simulink model "AEL_simple_model_v02"  (R2022b)
settings: Solver=FixedStepAuto  StartTime=0.0  StopTime=1  FixedStep=0.001  RelTol=1e-3  EnableMultiTasking=on
settings Model: Creator=Kumar  LastModifiedBy=Kumar
settings SolverCC: AllowMultiTaskInputOutput=on
settings DebuggingCC: MaxConsecutiveZCsMsg=none  ModelReferenceExtraNoncontSigs=none

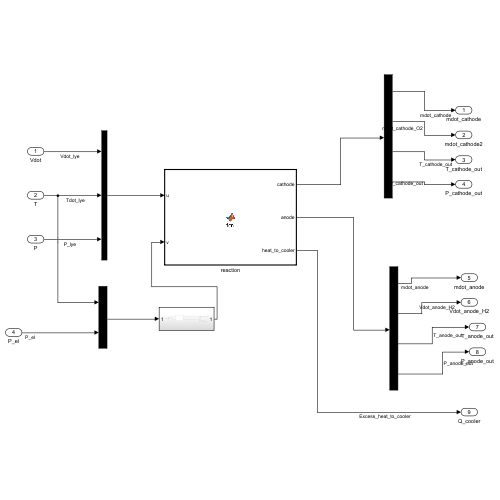
[thumbnail: Simulink's stored preview of the top-level diagram]
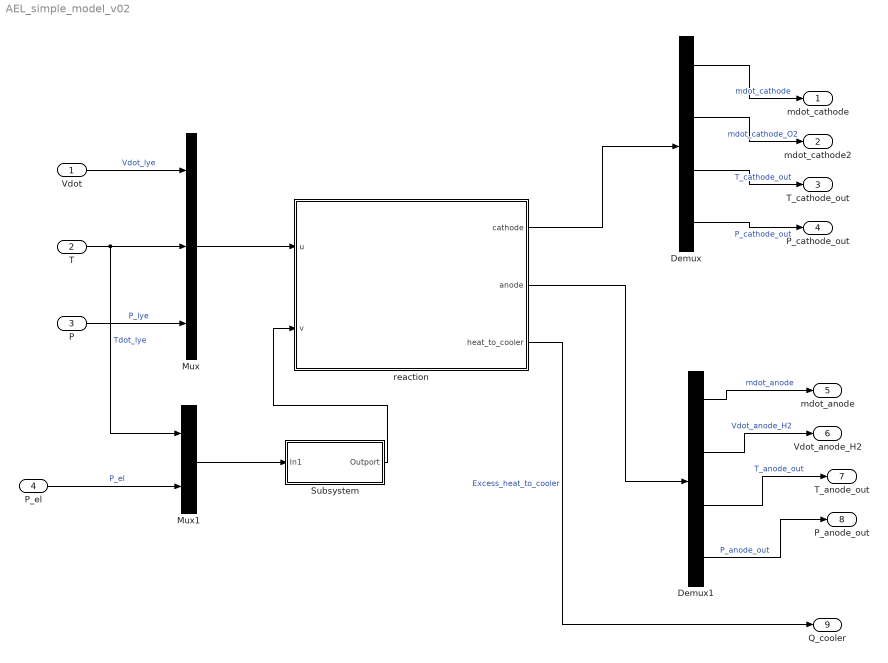
== system AEL_simple_model_v02 ==
  Vdot : Inport
  T : Inport  Port=2
  P : Inport  Port=3
  P_el : Inport  Port=4
  Demux : Demux
  Demux1 : Demux
  Mux : Mux  Inputs=3
  Mux1 : Mux  Inputs=2
  Subsystem : Subsystem
  reaction : MATLAB Function  TreatAsAtomicUnit=on
  mdot_cathode : Outport
  mdot_cathode2 : Outport  Port=2
  T_cathode_out : Outport  Port=3
  P_cathode_out : Outport  Port=4
  mdot_anode : Outport  Port=5
  Vdot_anode_H2 : Outport  Port=6
  T_anode_out : Outport  Port=7
  P_anode_out : Outport  Port=8
  Q_cooler : Outport  Port=9
  wires:
  Vdot/1 -> Mux/1  "Vdot_lye"
  Demux1/1 -> mdot_anode/1  "mdot_anode"
  T/1 -> Mux1/1, Mux/2  "Tdot_lye"
  Demux/1 -> mdot_cathode/1  "mdot_cathode"
  Mux/1 -> reaction/1(u)
  Demux1/2 -> Vdot_anode_H2/1  "Vdot_anode_H2"
  reaction/3(heat_to_cooler) -> Q_cooler/1  "Excess_heat_to_cooler"
  Mux1/1 -> Subsystem/1(In1)
  P/1 -> Mux/3  "P_lye"
  P_el/1 -> Mux1/2  "P_el"
  reaction/2(anode) -> Demux1/1
  Subsystem/1(Outport) -> reaction/2(v)
  reaction/1(cathode) -> Demux/1
  Demux/3 -> T_cathode_out/1  "T_cathode_out"
  Demux1/3 -> T_anode_out/1  "T_anode_out"
  Demux/4 -> P_cathode_out/1  "P_cathode_out"
  Demux/2 -> mdot_cathode2/1  "mdot_cathode_O2"
  Demux1/4 -> P_anode_out/1  "P_anode_out"

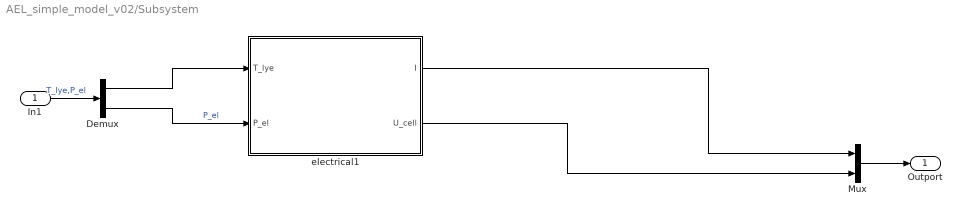
== system AEL_simple_model_v02/Subsystem ==
  In1 : Inport
  Demux : Demux  Outputs=2
  Mux : Mux  Inputs=2
  electrical1 : MATLAB Function  TreatAsAtomicUnit=on
  Outport : Outport
  wires:
  In1/1 -> Demux/1  "T_lye,P_el"
  Demux/1 -> electrical1/1(T_lye)
  Mux/1 -> Outport/1
  electrical1/1(I) -> Mux/1
  electrical1/2(U_cell) -> Mux/2
  Demux/2 -> electrical1/2(P_el)  "P_el"

== matlab function AEL_simple_model_v02/reaction ==
  data: u input; cathode output; anode output; heat_to_cooler output; v input
function [cathode, anode, heat_to_cooler] = fcn(u,v)

% Modelling assumptions: 
% 30% KOH solution
% Parameters

MwtH2 = 2.0; % Molecular weight of Hydrogen kg/kmol
MwtO2 = 32.0; % Molecular weight of Oxygen kg/kmol
MwtH2O = 18.0; % Molecular weight of water kg/kmol
z_value = 2; % Number of electrons transferred 
Farad = 96485000; % C/K mole Faraday's constant
param_d1 = -3.12996*10^-6; % Parameter from the polarization curve ohm m²
param_d2 = 4.47137 * 10^-7; % Parameter from the polarization curve ohm m² bar-1
A_electrode =  0.25; % Please note that the unit for current density is in m²
rho_lye = 1290; % Density of the KOH solution in kg/m³ --> Assumed constant 
n_c = 21; % No.of cells
R = 8.3144; % Gas constant KJ/KmolK
del_H0 = 286000; % standard enthalpy of reaction KJ/Kmol
T_amb = 298.15; % Ambient temperature - 25°C
Cp_lye = 4.2; % KJ/Kg K Specific heat capacity of lye --> assumed as that of water 

% Inputs

Vdot_lye = u(1) /(1000*3600); % volumetric flow of lye --> lph --> m³/s
T_lye = u(2); %353.75; % Temperature of lye K 
P_lye = u(3); %7.1  % Pressure of lye bar

I = v(1); % calculated current A/cm²
U_cell= v(2); % calculated voltage of cell V

% Equations

% Total electrode area
A = n_c * A_electrode; % m2 --> cm² needed

% Minimum reversible voltage
%U_rev = del_G/(z_value * Farad);

% Efficiency of the cell
yeta_f = 0.5; %(I/A)^2/(param_f1 + (I/A)^2) * param_f2; %0.86; %
% Mass balance
% Lye input at anode
mdot_anode_H2O = (Vdot_lye * rho_lye * 0.7) / 2; % kg/s
mdot_anode_KOH = (Vdot_lye * rho_lye * 0.3) / 2; % kg/s
ndot_anode_H2O = mdot_anode_H2O / MwtH2O; % kmol/s

% Lye input at cathode
mdot_cathode_H2O = (Vdot_lye * rho_lye* 0.7) / 2;  % kg/s
mdot_cathode_KOH = (Vdot_lye * rho_lye * 0.3) / 2;  % kg/s
ndot_cathode_H2O = mdot_cathode_H2O / MwtH2O;  % kmol/s

% Hydrogen produced at anode
ndot_anode_H2 = yeta_f * I /(z_value * Farad);% kmol/s
mdot_anode_H2 = ndot_anode_H2 * MwtH2; % kg/s
Vdot_anode_H2 = ndot_anode_H2 * 22.414; % Nm³/s

% Water going out of anode
ndot_anode_H2O_out = ndot_anode_H2O - ndot_anode_H2;% kmol/s
mdot_anode_H2O_out = ndot_anode_H2O_out * MwtH2O;% kg/s

% Oxygen produced at cathode
ndot_cathode_O2 = 0.5 * ndot_anode_H2; % kmol/s
mdot_cathode_O2 = ndot_cathode_O2 * MwtO2; % kg/s

% Water going out of anode
ndot_cathode_H2O_out = ndot_cathode_H2O + ndot_anode_H2; % kmol/s
mdot_cathode_H2O_out = ndot_cathode_H2O_out * MwtH2O; % kg/s

%Total flow out of cathode
%ndot_cathode = ndot_cathode_H2O_out + ndot_cathode_O2;
mdot_cathode = mdot_cathode_H2O_out + mdot_cathode_O2 + mdot_cathode_KOH; % kg/s
%Vdot_cathode = (mdot_cathode_H2O_out + mdot_cathode_KOH) / rho_lye + mdot_cathode_O2 / ((P_lye*10^5 * MwtO2)/(R *T_lye*1000)); 

% Total flow out of anode
%ndot_anode = ndot_anode_H2O_out + ndot_anode_H2;
mdot_anode = mdot_anode_H2O_out + mdot_anode_H2 + mdot_anode_KOH; % kg/s
%Vdot_anode = (mdot_anode_H2O_out + mdot_anode_KOH) / rho_lye + mdot_anode_H2 / ((P_lye*10^5 * MwtH2)/(R *T_lye*1000));

% Energy balance
% Calculating the del H for the process
del_H = del_H0 + Cp_lye*(T_lye-T_amb)*MwtH2O; %kJ/Kmol 

% Calculating the thermonuclear voltage
U_tn = del_H*1000 / (z_value * Farad); %V

% Heat generated in the process
Q_excess = I *(U_cell - U_tn); %KJ/s


% Outputs
cathode = [mdot_cathode*3600, mdot_cathode_O2*3600, T_lye, P_lye]
anode = [mdot_anode*3600, Vdot_anode_H2*3600, T_lye, P_lye]
heat_to_cooler = -Q_excess

== matlab function AEL_simple_model_v02/Subsystem/electrical1 ==
  data: T_lye input; P_el input; I output; U_cell output
function [ I, U_cell] = fcn(T_lye, P_el)

% Modelling assumptions: 
% Parameters
del_G = 237200.0; % KJ/Kmole Gibbs energy
Farad = 96485000; % C/Kmole Faraday's constant
param_t1 = -1.002; % m²/A co-effcient for overvoltage
param_t2 = 8.424; % m²°C/A co-effcient for overvoltage
param_t3 = 247.3; % m²°C²/A co-effcient for overvoltage
param_r1 = 8.05e-5; % ohm.m² ohmic resistance parameter
param_r2 = -2.5e-7; % ohm.m² ohmic resistance parameter
z_value = 2; % Number of electrons transferred
s = 0.185; 
%A_electrode = 0.25; %1000;  cm² Area of the cell l_c * w_c 21 * 0,25 (PHOEBUS)
%n_c = 12; % No.of cells

% Inputs T_lye and P_el
T = 75;%T_lye - 273.15; % °C
P_el = 10000;%P_el;
% Equations

% Total electrode area
A = 0.25*21; %n_c * A_electrode;

% Minimum reversible voltage
U_rev = del_G/(z_value * Farad);
r = param_r1 + param_r2*T ;
t = (param_t1 + param_t2/T + param_t3/T^2);

feq = @(x)[x(1) - P_el/x(2); x(2) - U_rev - s*log(abs(t * x(1)/A + 1)) - r*x(1)/A];
x0 = [8000, 1.3];
options = optimoptions('fsolve', 'Algorithm','levenberg-marquardt');
x = fsolve(feq, x0, options);

I = x(1)
U_cell = x(2)


% Efficiency of the cell
%yeta_f = 0.86; %(I/A)^2/(param_f1 + (I/A)^2) * param_f2; %0.86; %
